simulink subsystem "AdaptivePace"  (R2020a)
settings: Solver=VariableStepAuto  StartTime=0.0  StopTime=10.0  RelTol=1e-3
libraries: frdmk64flib x1
settings Model: Creator=amrad  LastModifiedBy=iceca

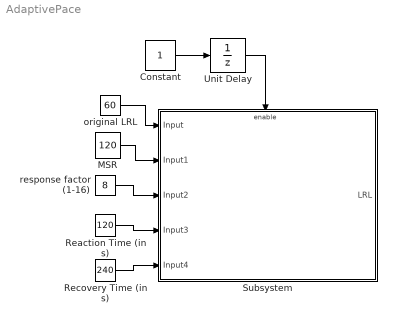
== system AdaptivePace ==
  Constant : Constant  OutDataTypeStr=boolean  SampleTime=0.1
  MSR : Constant  Value=120
  Reaction Time (in s) : Constant  Value=120
  Recovery Time (in s) : Constant  Value=240
  Subsystem : Subsystem
  Unit Delay : UnitDelay  SampleTime=-1  HasFrameUpgradeWarning=on
  original LRL : Constant  Value=60
  response factor (1-16) : Constant  Value=8
  wires:
  original LRL/1 -> Subsystem/1(Input)
  MSR/1 -> Subsystem/2(Input1)
  response factor (1-16)/1 -> Subsystem/3(Input2)
  Constant/1 -> Unit Delay/1
  Unit Delay/1 -> Subsystem/Enable
  Recovery Time (in s)/1 -> Subsystem/5(Input4)
  Reaction Time (in s)/1 -> Subsystem/4(Input3)

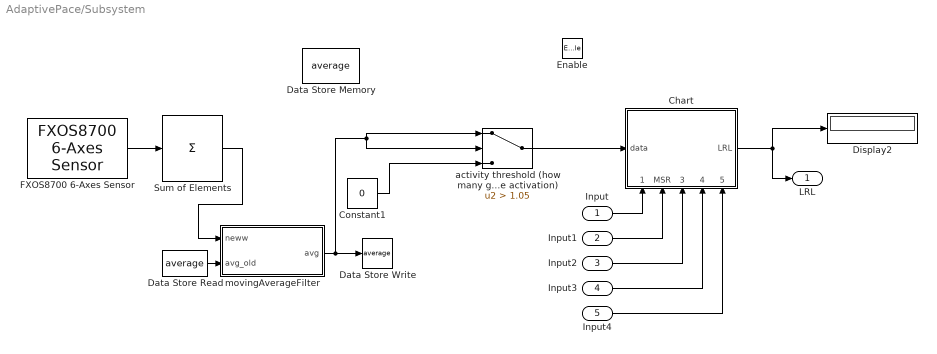
== system AdaptivePace/Subsystem ==
  Input : Inport
  Input1 : Inport  Port=2
  Input2 : Inport  Port=3
  Input3 : Inport  Port=4
  Input4 : Inport  Port=5
  Enable : EnablePort
  Chart : Stateflow chart  TreatAsAtomicUnit=on
      settings: PortSchema="{\"entries\":[{\"content\":{\"sides\":[{\"content\":{\"connectorIds\":[\"In6\"]},\"type\":\"ConnectorPlacement.EquallySpacedRectSide\",\"uuid\":\"5e590210-4b26-43ca-b410-899265592776\"},{\"content\":{\"connectorIds\":[\"Out1\"],\"side\":\"RIGHT\"},\"type\":\"ConnectorPlacement.EquallySpacedRectSide\",\"uuid\":\"99d9f5d1-b5a6-4f8b-b4f2-efe260ebc8c4\"},{\"content\":{\"connectorIds\":[],\"side\":\"TOP\"},\"type\":\"ConnectorPlacement.EquallySpacedRectSide\",\"uuid\":\"3c56162d-1f91-43ab-bf8d-9a1cf5be554c\"},{\"content\":{\"connectorIds\":[\"In1\",\"In2\",\"In3\",\"In4\",\"In5\"],\"side\":\"BOTTOM\"},\"type\":\"ConnectorPlacement.EquallySpacedRectSide\",\"uuid\":\"2e827a33-e1bf-40db-bbb6-314ece1f4eba\"}]},\"type\":\"ConnectorPlacement.EquallySpacedConnector\",\"uuid\":\"7a7dbe64-1607-48a8-bc2e-dcaf5b987588\"}],\"packageUris\":[\"http://schema.mathworks.com/mf0/Connector/19700101\"],\"version\":\"1.0\"}"
  Constant1 : Constant  Value=0  OutDataTypeStr=uint8
  Data Store Memory : DataStoreMemory  DataStoreName=average  ReadBeforeWriteMsg=warning  WriteAfterWriteMsg=warning  WriteAfterReadMsg=warning  ShowAdditionalParam=off
  Data Store Read : DataStoreRead  DataStoreName=average
  Data Store Write : DataStoreWrite  DataStoreName=average
  Display2 : Display
  FXOS8700 6-Axes Sensor : frdmk64flib/FXOS8700 6-Axes Sensor  Activesensor=Accelerometer only  ODR=800Hz  HybridODR=400Hz  Accelfullrange=-4g to +4g  SampleTime=-1
  Sum of Elements : Sum  Inputs=+
  activity threshold (how many gs before activation) : Switch  Criteria=u2 > Threshold  Threshold=1.05
  movingAverageFilter : MATLAB Function  TreatAsAtomicUnit=on
  LRL : Outport
  wires:
  FXOS8700 6-Axes Sensor/1 -> Sum of Elements/1
  Sum of Elements/1 -> movingAverageFilter/1(neww)
  Input2/1 -> Chart/3(ResponseFactor)
  Input1/1 -> Chart/2(MSR)
  Constant1/1 -> activity threshold (how many gs before activation)/3
  Chart/1(LRL) -> Display2/1, LRL/1
  Input/1 -> Chart/1(OLRL)
  activity threshold (how many gs before activation)/1 -> Chart/6(data)
  movingAverageFilter/1(avg) -> activity threshold (how many gs before activation)/2, activity threshold (how many gs before activation)/1, Data Store Write/1
  Input3/1 -> Chart/4(reactionTime)
  Input4/1 -> Chart/5(recoveryTime)
  Data Store Read/1 -> movingAverageFilter/2(avg_old)

== matlab function AdaptivePace/Subsystem/movingAverageFilter ==
  data: neww input; avg output; avg_old input
function avg = fcn(neww, avg_old)

avg = 0.9*avg_old+0.1*neww;

== stateflow chart AdaptivePace/Subsystem/Chart ==
  state start
    entry:
    LRL=OLRL
    RateChange=ResponseFactor/16
    diff=MSR-OLRL/RateChange
    reactionTick=reactionTime*1000/diff
    recoveryTick=recoveryTime*1000/diff
  state main
    entry:
  state Decreasing
    entry:
    LRL=LRL-RateChange
  state Increasing
    entry:
    LRL=LRL+RateChange
  (default) -> start
  start -> main
  main -> Decreasing [order 1] : [data==0 && LRL>OLRL]
  main -> Increasing [order 2] : [data>0 && LRL<MSR]
  Increasing -> main : [after(reactionTick,msec)]
  Decreasing -> main : [after(recoveryTick,msec)]
  data: OLRL input; MSR input; ResponseFactor input; reactionTime input; recoveryTime input; data input; LRL output double; RateChange local; recoveryTick local; reactionTick local; diff local
